simulink model "Sim_Helikopter_vereinfacht"  (R2015b)
settings: Solver=ode113  StartTime=0.0  StopTime=100  RelTol=1e-3
InitFcn:
  | Initialisierung
values from neighbouring files (symbols this model uses):
  q10e = 0    [Initialisierung.m]
  q1d = 2*pi    (= 6.28318530718)    [Initialisierung.m]
  q20e = 0.319187912478128    (= 0.319187912478)    [Initialisierung.m]
  q2d = 0    [Initialisierung.m]
  sysPar = block.DialogPrm(1).Data    [ROFLcopter_modell_S.m]
settings Model: Creator=Daniel  LastModifiedBy=danielhauer

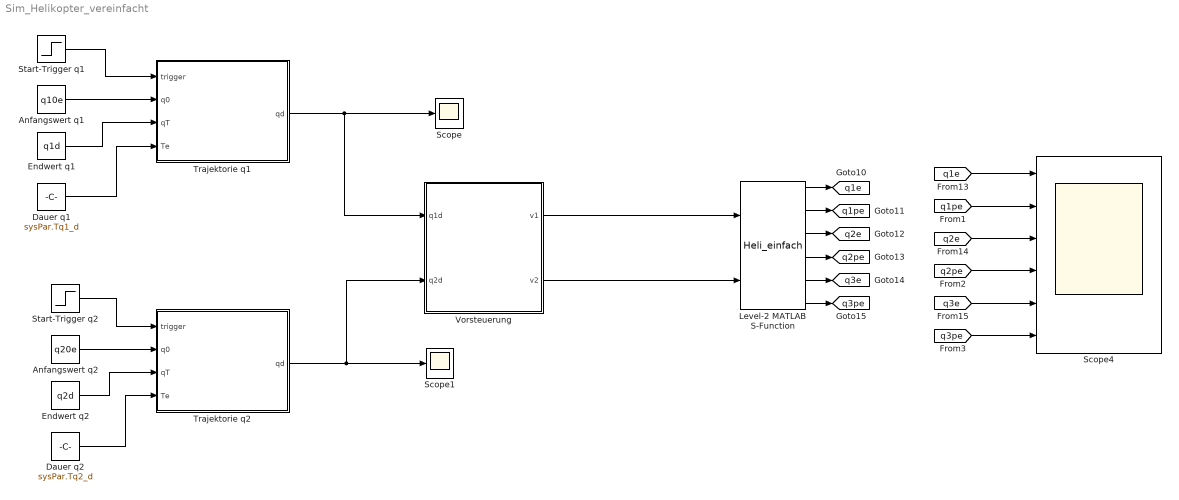
== system Sim_Helikopter_vereinfacht ==
  Anfangswert q1 : Constant  Value=q10e
  Anfangswert q2 : Constant  Value=q20e
  Dauer q1 : Constant  Value=sysPar.Tq1_d
  Dauer q2 : Constant  Value=sysPar.Tq2_d
  Endwert q1 : Constant  Value=q1d
  Endwert q2 : Constant  Value=q2d
  Level-2 MATLAB S-Function : M-S-Function  FunctionName=Heli_einfach  Parameters=sysPar.xR [sysPar.a1 sysPar.a2 sysPar.a3 sysPar.b1 sysPar.b2 sysPar.b3]
  Scope : Scope
  Scope1 : Scope
  Scope4 : Scope  NumInputPorts=6
  Start-Trigger q1 : Step  Time=sysPar.Tq1_s  SampleTime=0
  Start-Trigger q2 : Step  Time=sysPar.Tq2_s  SampleTime=0
  Trajektorie q1 : MATLAB Function  TreatAsAtomicUnit=on
  Trajektorie q2 : MATLAB Function  TreatAsAtomicUnit=on
  "Vorsteuerung " : MATLAB Function  TreatAsAtomicUnit=on
  tag scope: q1e=global, q1pe=global, q2e=global, q2pe=global, q3e=global, q3pe=global
  wires:
  Level-2 MATLAB S-Function/6 -> [q3pe]
  Level-2 MATLAB S-Function/5 -> [q3e]
  Level-2 MATLAB S-Function/4 -> [q2pe]
  Level-2 MATLAB S-Function/3 -> [q2e]
  Level-2 MATLAB S-Function/2 -> [q1pe]
  Level-2 MATLAB S-Function/1 -> [q1e]
  [q3e] -> Scope4/5
  [q2e] -> Scope4/3
  [q1e] -> Scope4/1
  Start-Trigger q1/1 -> Trajektorie q1/1(trigger)
  Anfangswert q1/1 -> Trajektorie q1/2(q0)
  Endwert q1/1 -> Trajektorie q1/3(qT)
  Start-Trigger q2/1 -> Trajektorie q2/1(trigger)
  Anfangswert q2/1 -> Trajektorie q2/2(q0)
  Endwert q2/1 -> Trajektorie q2/3(qT)
  [q1pe] -> Scope4/2
  [q2pe] -> Scope4/4
  [q3pe] -> Scope4/6
  Trajektorie q1/1(qd) -> "Vorsteuerung "/1(q1d), Scope/1
  Dauer q2/1 -> Trajektorie q2/4(Te)
  Dauer q1/1 -> Trajektorie q1/4(Te)
  "Vorsteuerung "/1(v1) -> Level-2 MATLAB S-Function/1
  "Vorsteuerung "/2(v2) -> Level-2 MATLAB S-Function/2
  Trajektorie q2/1(qd) -> "Vorsteuerung "/2(q2d), Scope1/1

== matlab function Sim_Helikopter_vereinfacht/Trajektorie q1 ==
  settings: updateMethod=DISCRETE  sampleTime=Ta
  data: trigger input; qd output; q0 input; qT input; Te input; sysPar parameter
function qd  = fcn(trigger,q0,qT,Te,sysPar)


beta5 = sysPar.beta5;
beta6 = sysPar.beta6;
beta7 = sysPar.beta7;
beta8 = sysPar.beta8;
beta9 = sysPar.beta9;


persistent t;

Ta=sysPar.Ta;
T=Te;
if isempty(t)
    t=0;
end
if(trigger)
    q=q0 + (qT-q0) * (beta5*(t/T)^5+beta6*(t/T)^6+beta7*(t/T)^7+beta8*(t/T)^8+beta9*(t/T)^9);
    qp=(qT - q0) * (5 * beta5 * t ^ 4 / T ^ 5 + 6 * beta6 * t ^ 5 / T ^ 6 + 7 * beta7 * t ^ 6 / T ^ 7 + 8 * beta8 * t ^ 7 / T ^ 8 + 9 * beta9 * t ^ 8 / T ^ 9);
    qpp=(qT - q0) * (20 * beta5 * t ^ 3 / T ^ 5 + 30 * beta6 * t ^ 4 / T ^ 6 + 42 * beta7 * t ^ 5 / T ^ 7 + 56 * beta8 * t ^ 6 / T ^ 8 + 72 * beta9 * t ^ 7 / T ^ 9);
    qppp=(qT - q0) * (60 * beta5 * t ^ 2 / T ^ 5 + 120 * beta6 * t ^ 3 / T ^ 6 + 210 * beta7 * t ^ 4 / T ^ 7 + 336 * beta8 * t ^ 5 / T ^ 8 + 504 * beta9 * t ^ 6 / T ^ 9); 
    qpppp=(qT - q0) * (120 * beta5 * t / T ^ 5 + 360 * beta6 * t ^ 2 / T ^ 6 + 840 * beta7 * t ^ 3 / T ^ 7 + 1680 * beta8 * t ^ 4 / T ^ 8 + 3024 * beta9 * t ^ 5 / T ^ 9);

       
    if t<T
        t=t+Ta;
        qd=[q;qp;qpp;qppp;qpppp];
    else
        qd=[qT;0;0;0;0];  
    end
    
else
    qd=[q0;0;0;0;0];
end

== matlab function Sim_Helikopter_vereinfacht/Trajektorie q2 ==
  settings: updateMethod=DISCRETE  sampleTime=Ta
  data: trigger input; qd output; q0 input; qT input; Te input; sysPar parameter
function qd  = fcn(trigger,q0,qT,Te,sysPar)

beta5 = sysPar.beta5;
beta6 = sysPar.beta6;
beta7 = sysPar.beta7;
beta8 = sysPar.beta8;
beta9 = sysPar.beta9;


persistent t;

Ta=sysPar.Ta;
T=Te;
if isempty(t)
    t=0;
end
if(trigger)
    q=q0 + (qT-q0) * (beta5*(t/T)^5+beta6*(t/T)^6+beta7*(t/T)^7+beta8*(t/T)^8+beta9*(t/T)^9);
    qp=(qT - q0) * (5 * beta5 * t ^ 4 / T ^ 5 + 6 * beta6 * t ^ 5 / T ^ 6 + 7 * beta7 * t ^ 6 / T ^ 7 + 8 * beta8 * t ^ 7 / T ^ 8 + 9 * beta9 * t ^ 8 / T ^ 9);
    qpp=(qT - q0) * (20 * beta5 * t ^ 3 / T ^ 5 + 30 * beta6 * t ^ 4 / T ^ 6 + 42 * beta7 * t ^ 5 / T ^ 7 + 56 * beta8 * t ^ 6 / T ^ 8 + 72 * beta9 * t ^ 7 / T ^ 9);
    qppp=(qT - q0) * (60 * beta5 * t ^ 2 / T ^ 5 + 120 * beta6 * t ^ 3 / T ^ 6 + 210 * beta7 * t ^ 4 / T ^ 7 + 336 * beta8 * t ^ 5 / T ^ 8 + 504 * beta9 * t ^ 6 / T ^ 9); 
    qpppp=(qT - q0) * (120 * beta5 * t / T ^ 5 + 360 * beta6 * t ^ 2 / T ^ 6 + 840 * beta7 * t ^ 3 / T ^ 7 + 1680 * beta8 * t ^ 4 / T ^ 8 + 3024 * beta9 * t ^ 5 / T ^ 9);

       
    if t<=T
        t=t+Ta;
        qd=[q;qp;qpp;qppp;qpppp];
    else
        qd=[qT;0;0;0;0];  
    end
    
else
    qd=[q0;0;0;0;0];
end

== matlab function Sim_Helikopter_vereinfacht/Vorsteuerung  ==
  settings: updateMethod=DISCRETE  sampleTime=Ta
  data: q1d input; v1 output; q2d input; sysPar parameter; v2 output
function [v1,v2] = fcn(q1d,q2d,sysPar)

q1pp=q1d(3);
q1ppp=q1d(4);
q1pppp=q1d(5);

a1=sysPar.a1;
a2=sysPar.a2;
a3=sysPar.a3;
b1=sysPar.b1;
b2=sysPar.b2;
b3=sysPar.b3;

q2=q2d(1);
q2p=q2d(2);
q2pp=q2d(3);
q2ppp=q2d(4);
q2pppp=q2d(5);

v1 = -0.1e1 / b2 * (a1 * sin(q2) + a2 * cos(q2) - q2pp) * sqrt(b2 ^ 2 * q1pp ^ 2 / b1 ^ 2 / cos(q2) ^ 2 / (a1 * sin(q2) + a2 * cos(q2) - q2pp) ^ 2 + 0.1e1);
v2 = -(-a3 * b2 * q1pp / b1 / (a1 * sin(q2) + a2 * cos(q2) - q2pp) * (b2 ^ 2 * q1pp ^ 2 / b1 ^ 2 / cos(q2) ^ 2 / (a1 * sin(q2) + a2 * cos(q2) - q2pp) ^ 2 + 0.1e1) ^ (-0.1e1 / 0.2e1) - b2 * ((-a1 * sin(q2) - a2 * cos(q2) + q2pp) * cos(q2) * (b2 ^ 2 * q1pp ^ 2 + b1 ^ 2 * cos(q2) ^ 2 * (-a1 * sin(q2) - a2 * cos(q2) + q2pp) ^ 2) * q1pppp - q1pp * cos(q2) * (b2 ^ 2 * q1pp ^ 2 + b1 ^ 2 * cos(q2) ^ 2 * (-a1 * sin(q2) - a2 * cos(q2) + q2pp) ^ 2) * q2pppp - 0.2e1 * q1pp * b2 ^ 2 * cos(q2) * (-a1 * sin(q2) - a2 * cos(q2) + q2pp) * q1ppp ^ 2 - 0.2e1 * (b2 * q1pp - b1 * cos(q2) * (-a1 * sin(q2) - a2 * cos(q2) + q2pp)) * (-cos(q2) * q2ppp + q2p * (a1 * cos(q2) ^ 2 - a1 * sin(q2) ^ 2 - 0.2e1 * a2 * sin(q2) * cos(q2) + q2pp * sin(q2))) * (b2 * q1pp + b1 * cos(q2) * (-a1 * sin(q2) - a2 * cos(q2) + q2pp)) * q1ppp + q1pp * (0.2e1 * b1 ^ 2 * cos(q2) ^ 3 * (-a1 * sin(q2) - a2 * cos(q2) + q2pp) * q2ppp ^ 2 + 0.2e1 * (q1pp ^ 2 * b2 ^ 2 * sin(q2) - b1 ^ 2 * cos(q2) ^ 2 * (0.2e1 * a1 * cos(q2) ^ 2 - a1 * sin(q2) ^ 2 - 0.3e1 * a2 * sin(q2) * cos(q2) + q2pp * sin(q2)) * (-a1 * sin(q2) - a2 * cos(q2) + q2pp)) * q2p * q2ppp + (q2pp ^ 2 * sin(q2) + (q2p ^ 2 * cos(q2) + a1 * cos(q2) ^ 2 - a1 * sin(q2) ^ 2 - 0.2e1 * a2 * sin(q2) * cos(q2)) * q2pp - 0.4e1 * (a1 * cos(q2) * sin(q2) + a2 * cos(q2) ^ 2 / 0.2e1 - a2 * sin(q2) ^ 2 / 0.2e1) * q2p ^ 2) * b2 ^ 2 * q1pp ^ 2 + (q2pp ^ 3 * cos(q2) * sin(q2) + ((cos(q2) ^ 2 + 0.2e1 * sin(q2) ^ 2) * q2p ^ 2 + cos(q2) * (a1 * cos(q2) ^ 2 - 0.2e1 * a1 * sin(q2) ^ 2 - 0.3e1 * a2 * sin(q2) * cos(q2))) * q2pp ^ 2 + ((-a1 * cos(q2) ^ 2 * sin(q2) - 0.4e1 * a1 * sin(q2) ^ 3 - 0.3e1 * a2 * cos(q2) ^ 3 - 0.6e1 * a2 * cos(q2) * sin(q2) ^ 2) * q2p ^ 2 - cos(q2) * (a1 * cos(q2) ^ 2 - a1 * sin(q2) ^ 2 - 0.2e1 * a2 * sin(q2) * cos(q2)) * (a1 * sin(q2) + a2 * cos(q2))) * q2pp + 0.2e1 * ((a1 ^ 2 + a2 ^ 2) * cos(q2) ^ 4 - a1 * a2 * cos(q2) ^ 3 * sin(q2) + 0.3e1 * a2 ^ 2 * cos(q2) ^ 2 * sin(q2) ^ 2 + 0.3e1 * a1 * a2 * cos(q2) * sin(q2) ^ 3 + a1 ^ 2 * sin(q2) ^ 4) * q2p ^ 2) * (-a1 * sin(q2) - a2 * cos(q2) + q2pp) * cos(q2) * b1 ^ 2)) * b1 / (b2 ^ 2 * q1pp ^ 2 + b1 ^ 2 * cos(q2) ^ 2 * (-a1 * sin(q2) - a2 * cos(q2) + q2pp) ^ 2) ^ 2) / b3;
